simulink model "ACC"  (R2020a)
settings: Solver=ode1  StartTime=0.0  StopTime=30  FixedStep=0.01  RelTol=1e-3  EnableMultiTasking=on
PreLoadFcn:
  | % Ex12_5.m
  | g=9.81; uw=0.0; u0=30.0; rho=1.202; Theta=0.0; ThetaPrime=0.0;
  | %Controlled vehicle parameters:
  | mc=1000.0; Cdc=0.5; Arc=1.5; fc=0.015;
  | Kc=(1/(rho*Cdc*Arc*(u0+uw))); Tc=mc*Kc;
  | wc0=mc*g*(fc*sin(Theta)-cos(Theta))*ThetaPrime; Fc=(u0/Kc);
  | % Lead vehicle parameters(typical):
  | ml = 1500.0; Cdl=0.6; Arl=1.95; fl=0.015;
  | Kl=(1/(rho*Cdl*Arl*(u0+uw))); Tl=ml*Kl;
  | Fl=(u0/Kl);
  | wl0=(ml*g*(fl*sin(Theta)-cos(Theta))*ThetaPrime);
  | t=[0:0.1:20]';
  | U0=Fc*ones(size(t));	% Nominal control force
  | wl = -800*(1+0.01*t);
  | wc = wc0*ones(size(t));
  | disturbance=[U0 wc wl];
  | % 4-state system for controller-design:
  | Aa=[0 -1 0 0; 0 -1/Tc 0 0; 1 0 0 0; 0 0 1 0];
  | Ba=[0;Kc/Tc;0;0];
  | % Controller design:
  | pc = [roots([1 2*0.9*0.4 0.4^2]); -1.08; -1.18];
  | K = place(Aa,Ba,pc); r0 = 30;
settings Model: Creator=경조  LastModifiedBy=user
settings SolverCC: SolverJacobianMethodControl=FullAnalytical
settings DataIOCC: ExternalInput=r  LimitDataPoints=on  SaveFormat=Array  SignalLoggingSaveFormat=ModelDataLogs  ReturnWorkspaceOutputs=off
settings OptimizationCC: ExpressionDepthLimit=2147483647  LifeSpan=1  EfficientTunableParamExpr=on
settings DebuggingCC: UnderspecifiedInitializationDetection=Classic  MergeDetectMultiDrivingBlocksExec=none  SolverPrmCheckMsg=warning  MultiTaskDSMMsg=warning  MultiTaskCondExecSysMsg=none  FcnCallInpInsideContextMsg=warning  StateNameClashWarn=warning  SFUnexpectedBacktrackingDiag=warning  SFNoUnconditionalDefaultTransitionDiag=warning  SFExecutionAtInitializationDiag=none  ArithmeticOperatorsInVariantConditions=warning
settings HardwareCC: ProdBitPerPointer=32  ProdBitPerSizeT=32  ProdBitPerPtrDiffT=32  ProdLargestAtomicFloat=None  ProdIntDivRoundTo=Undefined  ProdEndianess=Unspecified  ProdWordSize=32  ProdHWDeviceType=Generic->32-bit Embedded Processor
settings ModelReferenceCC: PropagateSignalLabelsOutOfModel=off
settings SFSimCC: SimUseLocalCustomCode=off  MATLABDynamicMemAlloc=off  CustomCodeUndefinedFunction=UseInterfaceOnly
settings RTWCC: SystemTargetFile=ert.tlc  TemplateMakefile=ert_default_tmf  RTWUseLocalCustomCode=off  RTWCompilerOptimization=on
settings CodeAppCC: IgnoreCustomStorageClasses=off  StateflowObjectComments=on
settings ERTTargetCC: MultiwordLength=2048  GenerateSampleERTMain=on  SupportContinuousTime=on  ERTCustomFileTemplate=example_file_process.tlc  ConvertIfToSwitch=off  SuppressUnreachableDefaultCases=off
settings ConfigComp: CovMetricSettings=dw  CovHtmlReporting=on  CovSaveCumulativeToWorkspaceVar=on  CovSaveSingleToWorkspaceVar=on  CovExternalEMLEnable=off

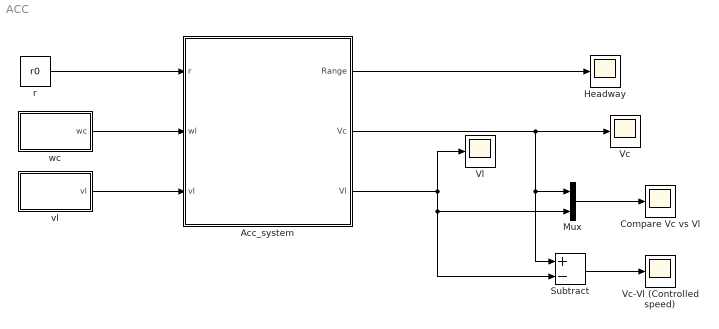
== system ACC ==
  Acc_system : Subsystem
  Compare Vc vs Vl : Scope
  Headway : Scope
  Mux : Mux  Inputs=2
  Subtract : Sum  Inputs=+-
  Vc : Scope
  Vc-Vl (Controlled speed) : Scope
  Vl : Scope
  r : Constant  Value=r0
  vl : Subsystem
  wc : Subsystem
  wires:
  r/1 -> Acc_system/1(r)
  vl/1(vl) -> Acc_system/3(vl)
  wc/1(wc) -> Acc_system/2(wl)
  Acc_system/1(Range) -> Headway/1
  Acc_system/2(Vc) -> Vc/1, Subtract/1, Mux/1
  Acc_system/3(Vl) -> Vl/1, Subtract/2, Mux/2
  Mux/1 -> Compare Vc vs Vl/1
  Subtract/1 -> Vc-Vl (Controlled speed)/1

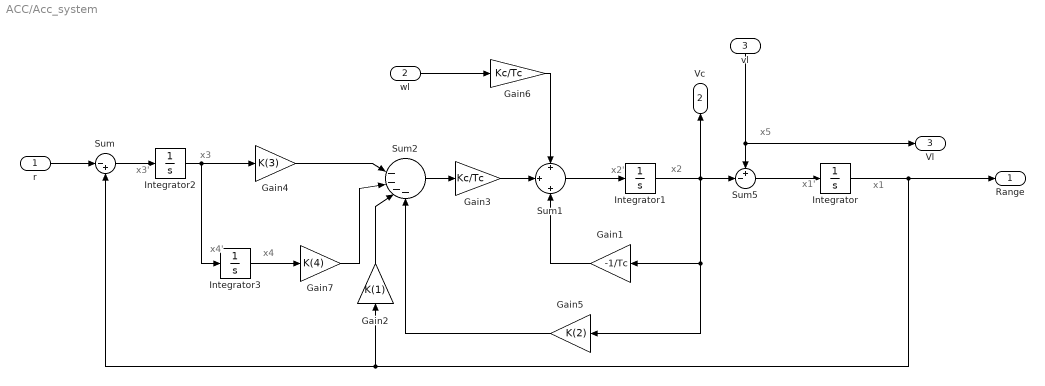
== system ACC/Acc_system ==
  note: x3'
  note: x3
  note: x4'
  note: x4
  note: x2'
  note: x1
  note: x2
  note: x5
  note: x1'
  r : Inport
  wl : Inport  Port=2
  vl : Inport  Port=3
  Gain1 : Gain  Gain=-1/Tc
  Gain2 : Gain  Gain=K(1)
  Gain3 : Gain  Gain=Kc/Tc
  Gain4 : Gain  Gain=K(3)
  Gain5 : Gain  Gain=K(2)
  Gain6 : Gain  Gain=Kc/Tc
  Gain7 : Gain  Gain=K(4)
  Integrator : Integrator  InitialCondition=r0
  Integrator1 : Integrator  InitialCondition=u0
  Integrator2 : Integrator
  Integrator3 : Integrator  InitialCondition=-(u0/Kc+K(1)*r0+K(2)*u0)/K(4)
  Sum : Sum  Inputs=|-+
  Sum1 : Sum  Inputs=+|+|+
  Sum2 : Sum  Inputs=||----
  Sum5 : Sum  Inputs=+-|
  Range : Outport
  Vc : Outport  Port=2
  Vl : Outport  Port=3
  wires:
  Sum5/1 -> Integrator/1
  Gain2/1 -> Sum2/3
  Sum/1 -> Integrator2/1
  Integrator/1 -> Range/1, Gain2/1, Sum/2
  Gain7/1 -> Sum2/2
  r/1 -> Sum/1
  Integrator1/1 -> Gain1/1, Gain5/1, Vc/1, Sum5/2
  Gain5/1 -> Sum2/4
  Sum1/1 -> Integrator1/1
  wl/1 -> Gain6/1
  Gain6/1 -> Sum1/1
  Integrator2/1 -> Integrator3/1, Gain4/1
  Gain4/1 -> Sum2/1
  Integrator3/1 -> Gain7/1
  vl/1 -> Vl/1, Sum5/1
  Gain1/1 -> Sum1/3
  Sum2/1 -> Gain3/1
  Gain3/1 -> Sum1/2

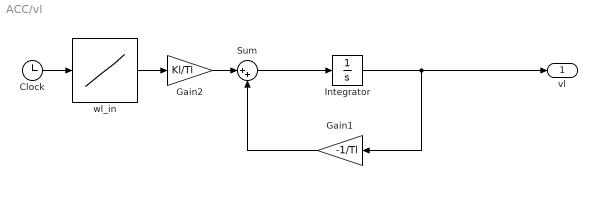
== system ACC/vl ==
  Clock : Clock
  Gain1 : Gain  Gain=-1/Tl
  Gain2 : Gain  Gain=Kl/Tl
  Integrator : Integrator  InitialCondition=u0
  Sum : Sum  Inputs=|++
  wl_in : Lookup_n-D  NumberOfTableDimensions=1  BreakpointsForDimension1=[0:0.1:20]  Table=wl  RndMeth=Simplest  InputSameDT=on
  vl : Outport
  wires:
  Integrator/1 -> vl/1, Gain1/1
  Gain1/1 -> Sum/2
  Sum/1 -> Integrator/1
  Clock/1 -> wl_in/1
  Gain2/1 -> Sum/1
  wl_in/1 -> Gain2/1

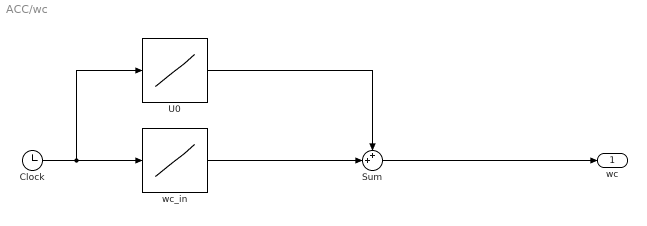
== system ACC/wc ==
  Clock : Clock
  Sum : Sum  Inputs=++|
  U0 : Lookup_n-D  NumberOfTableDimensions=1  BreakpointsForDimension1=[0:0.1:20]  Table=U0  RndMeth=Simplest  InputSameDT=on
  wc_in : Lookup_n-D  NumberOfTableDimensions=1  BreakpointsForDimension1=[0:0.1:20]  Table=wc  RndMeth=Simplest  InputSameDT=on
  wc : Outport
  wires:
  Clock/1 -> U0/1, wc_in/1
  U0/1 -> Sum/1
  Sum/1 -> wc/1
  wc_in/1 -> Sum/2
